simulink model "N3_Test"  (R2014b)
settings: Solver=ode3  SolverMode=SingleTasking  StartTime=0.0  StopTime=1e-4  FixedStep=fpgaclk  RelTol=1e-3
PreLoadFcn:
  | %fpgaclk=1/32.768e6
  | fpgaclk=1/49.152e6
  | 
  | SerialData=[1,zeros(1,11),1,0,0,1]
  | load ../window
  | win=win'   %Go back to using flatter and wider windowed sync function
  | %load ../hanning    %use Hahn window
  | 
  | load ../PREemphasis   %For pre-empasis and deemphasis FIRs
  | 
  | %LUT3=xls2LUT2('../IQI_Qdemod.xls'); LUT3
  | load ../LUT3
  | load ../FIRiq2
  | % xls2LUT
  | 
  | GetProgFiles
  | 
  | PinAssignments    %Get Pin references for TE0722
  | 
  | 
  | 
  | 
  | 
  | %LCD
  | LCDdata=[LCD_D7,LCD_D6,LCD_D5,LCD_D4,LCD_D3,LCD_D2,LCD_D1,LCD_D0] %Note MSB...LSB!
  | LCDctrl=[LCD_E,LCD_RW,LCD_RS];
  | 
  | %for RS232 on pins 3 and 5 of USBB
  | 
  | %BT chip connections for WT12
  | 
  | RX_BT=RXD
  | TX_BT=TXD
  | 
  | RST_BB=RES
  | 
  | %PCMC=PCMC
  | %PCMS=PCMS
  | %PCMI=PCMI
  | %PCMO=PCMO
  | 
  | %Aliases:
  | SRDBT=PCMI
  | STDBT=PCMO
  | SCLK_BT=PCMC
  | SFS_BT=PCMS
  | 
  | %ADC control
  | 
  | %SDOA=SDOA
  | %SDOB=SDOB
  | %SCK=SCK
  | CONV=Csbar
  | CAL=Cal
  | 
  | ADC_G=[ADC_G3,ADC_G2,ADC_G1,ADC_G0]
  | %PD settings hard coded now
  | 
  | %%%%%%
  | TX_LOW=TX_Low
  | 
  | %Leds
  | %Defined inPinassignments
  | 
  | 
  | 
  | %TouchPads
  | %Defined in Pinassignments
  | 
  | 
  | 'Got to end of pre-load OK'
StartFcn:
  | fpgaclk=1/32.768e6
  | SerialData=[1,zeros(1,11),1,0,0,1]
values from neighbouring files (symbols this model uses):
  ADC_G0 = {'P10'}    [PinAssignments.m]
  ADC_G1 = {'P11'}    [PinAssignments.m]
  ADC_G2 = {'N14'}    [PinAssignments.m]
  ADC_G3 = {'M11'}    [PinAssignments.m]
  Cal = {'L12'}    [PinAssignments.m]
  Csbar = {'M12'}    [PinAssignments.m]
  LCD_D0 = {'J13'}    [PinAssignments.m]
  LCD_D1 = {'J14'}    [PinAssignments.m]
  LCD_D2 = {'F15'}    [PinAssignments.m]
  LCD_D3 = {'H14'}    [PinAssignments.m]
  LCD_D4 = {'G12'}    [PinAssignments.m]
  LCD_D5 = {'L15'}    [PinAssignments.m]
  LCD_D6 = {'M14'}    [PinAssignments.m]
  LCD_D7 = {'K15'}    [PinAssignments.m]
  PCMC = {'H11'}    [PinAssignments.m]
  PCMI = {'H12'}    [PinAssignments.m]
  PCMO = {'N13'}    [PinAssignments.m]
  PCMS = {'M10'}    [PinAssignments.m]
  RES = {'G11'}    [PinAssignments.m]
  RXD = {'H13'}    [PinAssignments.m]
  TX_Low = {'P15'}    [PinAssignments.m]
  TXD = {'P13'}    [PinAssignments.m]
libraries: xbsIndex_r4 x8
settings Model: Creator=Graham  LastModifiedBy=graham
settings DataIOCC: SignalLoggingSaveFormat=ModelDataLogs  SignalLoggingName=sigsOut
settings OptimizationCC: ExpressionDepthLimit=2147483647  InitFltsAndDblsToZero=on
settings DebuggingCC: SaveWithParameterizedLinksMsg=none  UnderspecifiedInitializationDetection=Classic  MergeDetectMultiDrivingBlocksExec=none  SignalResolutionControl=TryResolveAllWithWarning  SolverPrmCheckMsg=none  MultiTaskDSMMsg=warning  MultiTaskCondExecSysMsg=none  StateNameClashWarn=warning
settings HardwareCC: TargetUnknown=on
settings RTWCC: IncludeERTFirstTime=on
settings GRTTargetCC: TargetFcnLib=ansi_tfl_tmw.mat  ModelReferenceCompliant=off  CombineOutputUpdateFcns=off  MatFileLogging=off  GRTInterface=on

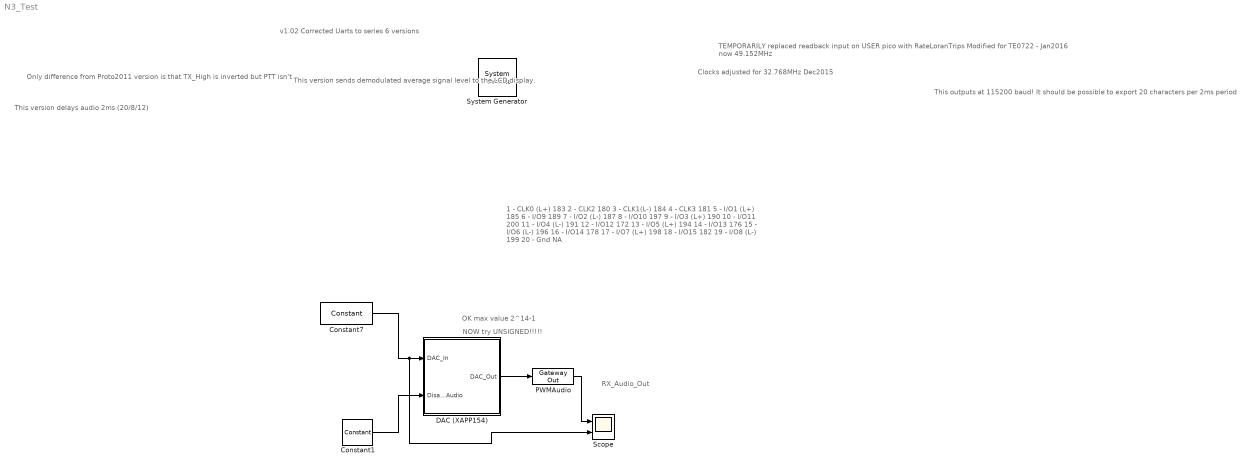
== system N3_Test ==
  note: v1.02 Corrected Uarts to series 6 versions
  note: OK max value 2^14-1
  note: This outputs at 115200 baud! It should be possible to export 20 characters per 2ms period
  note: 1 - CLK0 (L+)	183	2 - CLK2	180
      | 3 - CLK1(L-)	184	4 - CLK3	181
      | 5 - I/O1 (L+)	185	6 - I/O9	189
      | 7 - I/O2 (L-)	187	8 - I/O10	197
      | 9 - I/O3 (L+)	190	10 - I/O11	200
      | 11 - I/O4 (L-)	191	12 - I/O12	172
      | 13 - I/O5 (L+)	194	14 - I/O13	176
      | 15 - I/O6 (L-)	196	16 - I/O14	178
      | 17 - I/O7 (L+)	198	18 - I/O15	182
      | 19 - I/O8 (L-)	199	20 - Gnd	NA
  note: RX_Audio_Out
  note: Clocks adjusted for 32.768MHz Dec2015
  note: NOW try UNSIGNED!!!!!
  note: Only difference from Proto2011 version is that TX_High is inverted but PTT isn't
  note: This version delays audio 2ms (20/8/12)
  note: TEMPORARILY replaced readback input on USER pico with RateLoranTrips
      | Modified for TE0722 - Jan2016 now 49.152MHz
  note: This version sends demodulated average signal level to the LCD display.
  " System Generator" : xbsIndex_r4/ System Generator  Tag=genX  xilinxfamily=zynq  part=xc7z010  speed=-1  package=clg225  synthesis_tool=XST  clock_wrapper=Clock Enables  directory=../../SysgenOutput/TE0722  proj_type=Project Navigator  Synth_file=XST Defaults  Impl_file=ISE Defaults  testbench=off  simulink_period=fpgaclk  sysclk_period=30  dcm_input_clock_period=100  incr_netlist=off  trim_vbits=Everywhere in SubSystem  dbl_ovrd=According to Block Masks  core_generation=According to Block Masks  run_coregen=off  deprecated_control=off  eval_field=0  block_type=sysgen
      settings: block_version=8.2.02
  Constant1 : xbsIndex_r4/Constant  const=0  gui_display_data_type=Boolean  arith_type=Boolean  n_bits=16  bin_pt=0  preci_type=Single  exp_width=8  frac_width=24  explicit_period=on  period=fpgaclk  equ=P=C  opselect=C  inp2=PCIN>>17  opr=+  inp1=P  carry=CIN  dbl_ovrd=off  block_type=constant
      settings: block_version=VER_STRING_GOES_HERE
  Constant7 : xbsIndex_r4/Constant  const=2^12-1  gui_display_data_type=Fixed-point  arith_type=Unsigned  n_bits=14  bin_pt=0  preci_type=Single  exp_width=8  frac_width=24  explicit_period=on  period=fpgaclk  equ=P=C  opselect=C  inp2=PCIN>>17  opr=+  inp1=P  carry=CIN  dbl_ovrd=off  block_type=constant
      settings: block_version=VER_STRING_GOES_HERE
  DAC (XAPP154) : Subsystem
  PWMAudio : xbsIndex_r4/Gateway Out  inherit_from_input=off  hdl_port=on  rows=1  columns=1  UseAsDAC=off  DACChannel='1'  interface=None  automatic_assignment=on  address_offset=hex2dec('00')  intf_description=''  timing_constraint=None  locs_specified=on  LOCs=PWMAudio  io_standard={'LVCMOS33'}  block_type=gatewayout
      settings: xl_area=[0, 0, 0, 0, 0, 0, 0]  block_version=VER_STRING_GOES_HERE
  Scope : Scope  NumInputPorts=2
      settings: YMin=0~7782.4  YMax=1~8601.6
  wires:
  PWMAudio/1 -> Scope/1
  DAC (XAPP154)/1(DAC_Out) -> PWMAudio/1
  Constant1/1 -> DAC (XAPP154)/2(Disable_Audio)
  Constant7/1 -> Scope/2, DAC (XAPP154)/1(DAC_In)

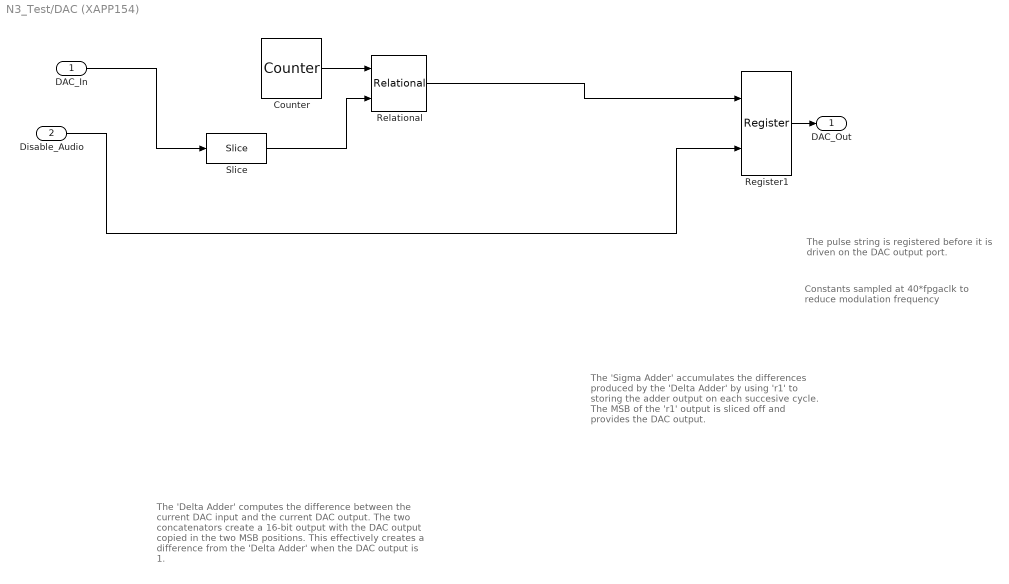
== system N3_Test/DAC (XAPP154) ==
  note: The 'Delta Adder' computes the difference
      | between the current DAC input and the current
      | DAC output.  The two concatenators create
      | a 16-bit output with the DAC output copied in the
      | two MSB positions. This effectively creates a
      | difference from the 'Delta Adder' when the DAC
      | output is 1.
  note: The 'Sigma Adder' accumulates the
      | differences produced by the 'Delta Adder'
      | by using 'r1' to storing the adder output on
      | each succesive cycle.  The MSB of the 'r1'
      | output is sliced off and provides the DAC
      | output.
  note: The pulse string is registered before
      | it is driven on the DAC output port.
  note: Constants sampled at 40*fpgaclk
      | to reduce modulation frequency
  DAC_In : Inport
  Disable_Audio : Inport  Port=2
  Counter : xbsIndex_r4/Counter  cnt_type=Free Running  cnt_to=Inf  operation=Up  start_count=0  cnt_by_val=1  arith_type=Unsigned  n_bits=8  bin_pt=0  load_pin=off  rst=off  en=off  explicit_period=on  period=fpgaclk  use_behavioral_HDL=off  implementation=Fabric  dbl_ovrd=off  block_type=counter
  Register1 : xbsIndex_r4/Register  init=0  rst=on  en=off  dbl_ovrd=off  block_type=register
      settings: xl_area=[1 1 0 0 0 0 0]  block_version=VER_STRING_GOES_HERE
  Relational : xbsIndex_r4/Relational  mode=a<b  op_type=Bool  en=off  latency=1  dbl_ovrd=off  block_type=relational
  Slice : xbsIndex_r4/Slice  nbits=8  boolean_output=off  mode=Upper Bit Location + Width  bit1=0  base1=MSB of Input  bit0=0  base0=LSB of Input  dbl_ovrd=off  block_type=slice
  DAC_Out : Outport
  wires:
  Register1/1 -> DAC_Out/1
  Disable_Audio/1 -> Register1/2
  DAC_In/1 -> Slice/1
  Counter/1 -> Relational/1
  Slice/1 -> Relational/2
  Relational/1 -> Register1/1
